simulink library "Snake_Lib"  (R2016a)
settings: Solver=ode45  StartTime=0.0  StopTime=10.0  RelTol=1e-3
libraries: Bit_Demultiplexers_Lib x5, Bit_Multiplexers_Lib x5, simulink_extras x5, commutil2 x2
settings Model: Creator=Jozko Mrkvicka  LastModifiedBy=Jozko Mrkvicka
settings DataIOCC: LimitDataPoints=on
settings DebuggingCC: AllowSymbolicDim=off

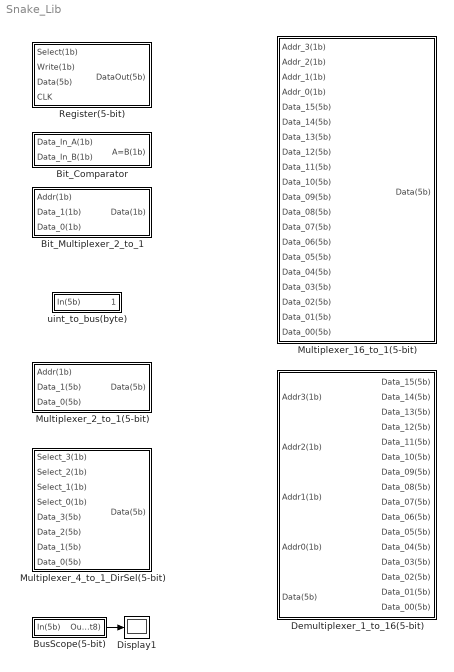
== system Snake_Lib ==
  Bit_Comparator : Subsystem
  Bit_Multiplexer_2_to_1 : Subsystem
  BusScope(5-bit) : Subsystem
  Demultiplexer_1_to_16(5-bit) : Subsystem
  Display1 : Display
  Multiplexer_16_to_1(5-bit) : Subsystem
  Multiplexer_2_to_1(5-bit) : Subsystem
  Multiplexer_4_to_1_DirSel(5-bit) : Subsystem
  Register(5-bit) : Subsystem
  uint_to_bus(byte) : Subsystem
  wires:
  BusScope(5-bit)/1(Out(int8)) -> Display1/1

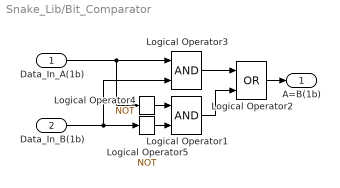
== system Snake_Lib/Bit_Comparator ==
  Data_In_A(1b) : Inport
  Data_In_B(1b) : Inport  Port=2
  Logical Operator1 : Logic  IconShape=distinctive  AllPortsSameDT=off  OutDataTypeStr=boolean
  Logical Operator2 : Logic  Operator=OR  IconShape=distinctive  AllPortsSameDT=off  OutDataTypeStr=boolean
  Logical Operator3 : Logic  IconShape=distinctive  AllPortsSameDT=off  OutDataTypeStr=boolean
  Logical Operator4 : Logic  Operator=NOT  IconShape=distinctive  AllPortsSameDT=off  OutDataTypeStr=boolean
  Logical Operator5 : Logic  Operator=NOT  IconShape=distinctive  AllPortsSameDT=off  OutDataTypeStr=boolean
  A=B(1b) : Outport
  wires:
  Logical Operator4/1 -> Logical Operator1/1
  Logical Operator3/1 -> Logical Operator2/1
  Logical Operator1/1 -> Logical Operator2/2
  Logical Operator2/1 -> A=B(1b)/1
  Data_In_A(1b)/1 -> Logical Operator4/1, Logical Operator3/1
  Logical Operator5/1 -> Logical Operator1/2
  Data_In_B(1b)/1 -> Logical Operator5/1, Logical Operator3/2

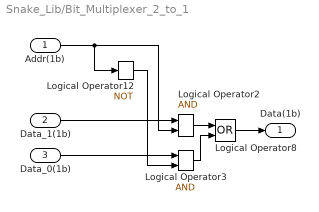
== system Snake_Lib/Bit_Multiplexer_2_to_1 ==
  Addr(1b) : Inport
  Data_1(1b) : Inport  Port=2
  Data_0(1b) : Inport  Port=3
  Logical Operator12 : Logic  Operator=NOT  Inputs=4  IconShape=distinctive  AllPortsSameDT=off  OutDataTypeStr=boolean
  Logical Operator2 : Logic  IconShape=distinctive  AllPortsSameDT=off  OutDataTypeStr=boolean
  Logical Operator3 : Logic  IconShape=distinctive  AllPortsSameDT=off  OutDataTypeStr=boolean
  Logical Operator8 : Logic  Operator=OR  IconShape=distinctive  OutDataTypeStr=boolean
  Data(1b) : Outport
  wires:
  Logical Operator2/1 -> Logical Operator8/1
  Logical Operator3/1 -> Logical Operator8/2
  Data_0(1b)/1 -> Logical Operator3/1
  Data_1(1b)/1 -> Logical Operator2/1
  Logical Operator8/1 -> Data(1b)/1
  Addr(1b)/1 -> Logical Operator12/1, Logical Operator2/2
  Logical Operator12/1 -> Logical Operator3/2

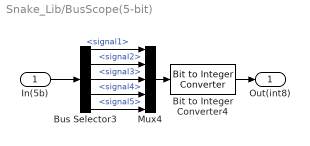
== system Snake_Lib/BusScope(5-bit) ==
  In(5b) : Inport
  Bit to Integer Converter4 : commutil2/Bit to Integer Converter  nbits=5  bitOrder=MSB first  signedOutputValues=Unsigned  outDtype=int8  outDtypeSigned=Inherit via internal rule
  Bus Selector3 : BusSelector  OutputSignals=signal1,signal2,signal3,signal4,signal5
  Mux4 : Mux  Inputs=5
  Out(int8) : Outport
  wires:
  Bus Selector3/2 -> Mux4/2  "<signal2>"
  Bus Selector3/3 -> Mux4/3  "<signal3>"
  Bus Selector3/4 -> Mux4/4  "<signal4>"
  Bus Selector3/5 -> Mux4/5  "<signal5>"
  Bus Selector3/1 -> Mux4/1  "<signal1>"
  Bit to Integer Converter4/1 -> Out(int8)/1
  In(5b)/1 -> Bus Selector3/1
  Mux4/1 -> Bit to Integer Converter4/1

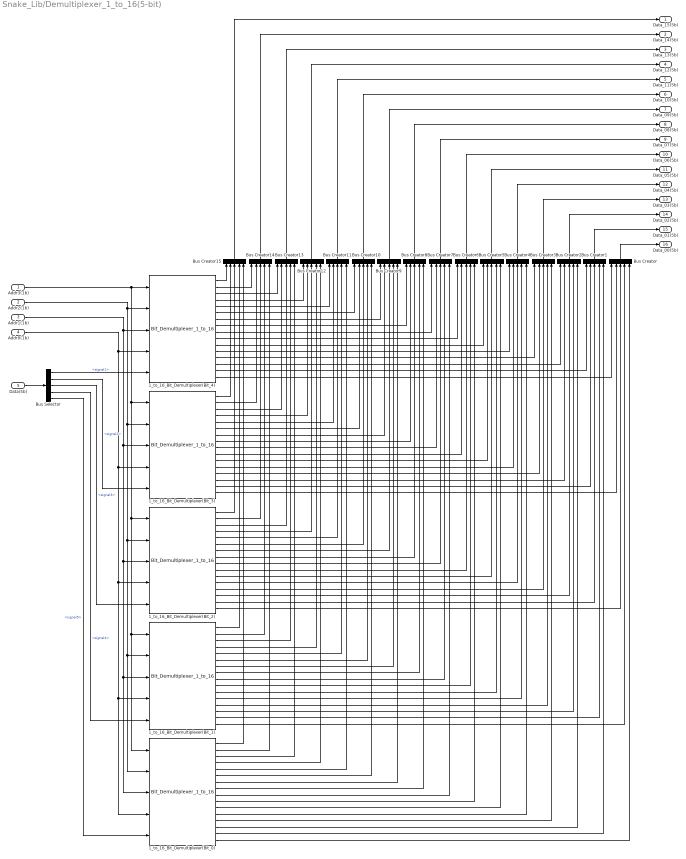
== system Snake_Lib/Demultiplexer_1_to_16(5-bit) ==
  Addr3(1b) : Inport
  Addr2(1b) : Inport  Port=2
  Addr1(1b) : Inport  Port=3
  Addr0(1b) : Inport  Port=4
  Data(5b) : Inport  Port=5
  1_to_16_Bit_Demultiplexer(Bit_0) : Bit_Demultiplexers_Lib/Bit_Demultiplexers_Lib/Bit_Demultiplexer_1_to_16
  1_to_16_Bit_Demultiplexer(Bit_1) : Bit_Demultiplexers_Lib/Bit_Demultiplexers_Lib/Bit_Demultiplexer_1_to_16
  1_to_16_Bit_Demultiplexer(Bit_2) : Bit_Demultiplexers_Lib/Bit_Demultiplexers_Lib/Bit_Demultiplexer_1_to_16
  1_to_16_Bit_Demultiplexer(Bit_3) : Bit_Demultiplexers_Lib/Bit_Demultiplexers_Lib/Bit_Demultiplexer_1_to_16
  1_to_16_Bit_Demultiplexer(Bit_4) : Bit_Demultiplexers_Lib/Bit_Demultiplexers_Lib/Bit_Demultiplexer_1_to_16
  Bus Creator{,1..15} (16 alike) : BusCreator  Inputs=5
  Bus Selector : BusSelector  OutputSignals=signal1,signal2,signal3,signal4,signal5
  Data_15(5b) : Outport
  Data_14(5b) : Outport  Port=2
  Data_13(5b) : Outport  Port=3
  Data_12(5b) : Outport  Port=4
  Data_11(5b) : Outport  Port=5
  Data_10(5b) : Outport  Port=6
  Data_09(5b) : Outport  Port=7
  Data_08(5b) : Outport  Port=8
  Data_07(5b) : Outport  Port=9
  Data_06(5b) : Outport  Port=10
  Data_05(5b) : Outport  Port=11
  Data_04(5b) : Outport  Port=12
  Data_03(5b) : Outport  Port=13
  Data_02(5b) : Outport  Port=14
  Data_01(5b) : Outport  Port=15
  Data_00(5b) : Outport  Port=16
  wires:
  Addr0(1b)/1 -> 1_to_16_Bit_Demultiplexer(Bit_4)/4, 1_to_16_Bit_Demultiplexer(Bit_0)/4, 1_to_16_Bit_Demultiplexer(Bit_1)/4, 1_to_16_Bit_Demultiplexer(Bit_2)/4, 1_to_16_Bit_Demultiplexer(Bit_3)/4
  Addr1(1b)/1 -> 1_to_16_Bit_Demultiplexer(Bit_4)/3, 1_to_16_Bit_Demultiplexer(Bit_0)/3, 1_to_16_Bit_Demultiplexer(Bit_1)/3, 1_to_16_Bit_Demultiplexer(Bit_2)/3, 1_to_16_Bit_Demultiplexer(Bit_3)/3
  Addr2(1b)/1 -> 1_to_16_Bit_Demultiplexer(Bit_4)/2, 1_to_16_Bit_Demultiplexer(Bit_0)/2, 1_to_16_Bit_Demultiplexer(Bit_1)/2, 1_to_16_Bit_Demultiplexer(Bit_2)/2, 1_to_16_Bit_Demultiplexer(Bit_3)/2
  Addr3(1b)/1 -> 1_to_16_Bit_Demultiplexer(Bit_0)/1, 1_to_16_Bit_Demultiplexer(Bit_1)/1, 1_to_16_Bit_Demultiplexer(Bit_2)/1, 1_to_16_Bit_Demultiplexer(Bit_3)/1, 1_to_16_Bit_Demultiplexer(Bit_4)/1
  Data(5b)/1 -> Bus Selector/1
  1_to_16_Bit_Demultiplexer(Bit_4)/1 -> Bus Creator15/1
  1_to_16_Bit_Demultiplexer(Bit_4)/2 -> Bus Creator14/1
  1_to_16_Bit_Demultiplexer(Bit_4)/3 -> Bus Creator13/1
  1_to_16_Bit_Demultiplexer(Bit_4)/4 -> Bus Creator12/1
  1_to_16_Bit_Demultiplexer(Bit_4)/5 -> Bus Creator11/1
  1_to_16_Bit_Demultiplexer(Bit_4)/6 -> Bus Creator10/1
  1_to_16_Bit_Demultiplexer(Bit_4)/7 -> Bus Creator9/1
  1_to_16_Bit_Demultiplexer(Bit_4)/8 -> Bus Creator8/1
  1_to_16_Bit_Demultiplexer(Bit_4)/9 -> Bus Creator7/1
  1_to_16_Bit_Demultiplexer(Bit_4)/10 -> Bus Creator6/1
  1_to_16_Bit_Demultiplexer(Bit_4)/11 -> Bus Creator5/1
  1_to_16_Bit_Demultiplexer(Bit_4)/12 -> Bus Creator4/1
  1_to_16_Bit_Demultiplexer(Bit_4)/13 -> Bus Creator3/1
  1_to_16_Bit_Demultiplexer(Bit_4)/14 -> Bus Creator2/1
  1_to_16_Bit_Demultiplexer(Bit_4)/15 -> Bus Creator1/1
  1_to_16_Bit_Demultiplexer(Bit_4)/16 -> Bus Creator/1
  1_to_16_Bit_Demultiplexer(Bit_3)/1 -> Bus Creator15/2
  1_to_16_Bit_Demultiplexer(Bit_3)/2 -> Bus Creator14/2
  1_to_16_Bit_Demultiplexer(Bit_3)/3 -> Bus Creator13/2
  1_to_16_Bit_Demultiplexer(Bit_3)/4 -> Bus Creator12/2
  1_to_16_Bit_Demultiplexer(Bit_3)/5 -> Bus Creator11/2
  1_to_16_Bit_Demultiplexer(Bit_3)/6 -> Bus Creator10/2
  1_to_16_Bit_Demultiplexer(Bit_3)/7 -> Bus Creator9/2
  1_to_16_Bit_Demultiplexer(Bit_3)/8 -> Bus Creator8/2
  1_to_16_Bit_Demultiplexer(Bit_3)/9 -> Bus Creator7/2
  1_to_16_Bit_Demultiplexer(Bit_3)/10 -> Bus Creator6/2
  1_to_16_Bit_Demultiplexer(Bit_3)/11 -> Bus Creator5/2
  1_to_16_Bit_Demultiplexer(Bit_3)/12 -> Bus Creator4/2
  1_to_16_Bit_Demultiplexer(Bit_3)/13 -> Bus Creator3/2
  1_to_16_Bit_Demultiplexer(Bit_3)/14 -> Bus Creator2/2
  1_to_16_Bit_Demultiplexer(Bit_3)/15 -> Bus Creator1/2
  1_to_16_Bit_Demultiplexer(Bit_3)/16 -> Bus Creator/2
  1_to_16_Bit_Demultiplexer(Bit_2)/1 -> Bus Creator15/3
  1_to_16_Bit_Demultiplexer(Bit_2)/2 -> Bus Creator14/3
  1_to_16_Bit_Demultiplexer(Bit_2)/3 -> Bus Creator13/3
  1_to_16_Bit_Demultiplexer(Bit_2)/4 -> Bus Creator12/3
  1_to_16_Bit_Demultiplexer(Bit_2)/5 -> Bus Creator11/3
  1_to_16_Bit_Demultiplexer(Bit_2)/6 -> Bus Creator10/3
  1_to_16_Bit_Demultiplexer(Bit_2)/7 -> Bus Creator9/3
  1_to_16_Bit_Demultiplexer(Bit_2)/8 -> Bus Creator8/3
  1_to_16_Bit_Demultiplexer(Bit_2)/9 -> Bus Creator7/3
  1_to_16_Bit_Demultiplexer(Bit_2)/10 -> Bus Creator6/3
  1_to_16_Bit_Demultiplexer(Bit_2)/11 -> Bus Creator5/3
  1_to_16_Bit_Demultiplexer(Bit_2)/12 -> Bus Creator4/3
  1_to_16_Bit_Demultiplexer(Bit_2)/13 -> Bus Creator3/3
  1_to_16_Bit_Demultiplexer(Bit_2)/14 -> Bus Creator2/3
  1_to_16_Bit_Demultiplexer(Bit_2)/15 -> Bus Creator1/3
  1_to_16_Bit_Demultiplexer(Bit_2)/16 -> Bus Creator/3
  1_to_16_Bit_Demultiplexer(Bit_1)/1 -> Bus Creator15/4
  1_to_16_Bit_Demultiplexer(Bit_1)/2 -> Bus Creator14/4
  1_to_16_Bit_Demultiplexer(Bit_1)/3 -> Bus Creator13/4
  1_to_16_Bit_Demultiplexer(Bit_1)/4 -> Bus Creator12/4
  1_to_16_Bit_Demultiplexer(Bit_1)/5 -> Bus Creator11/4
  1_to_16_Bit_Demultiplexer(Bit_1)/6 -> Bus Creator10/4
  1_to_16_Bit_Demultiplexer(Bit_1)/7 -> Bus Creator9/4
  1_to_16_Bit_Demultiplexer(Bit_1)/8 -> Bus Creator8/4
  1_to_16_Bit_Demultiplexer(Bit_1)/9 -> Bus Creator7/4
  1_to_16_Bit_Demultiplexer(Bit_1)/10 -> Bus Creator6/4
  1_to_16_Bit_Demultiplexer(Bit_1)/11 -> Bus Creator5/4
  1_to_16_Bit_Demultiplexer(Bit_1)/12 -> Bus Creator4/4
  1_to_16_Bit_Demultiplexer(Bit_1)/13 -> Bus Creator3/4
  1_to_16_Bit_Demultiplexer(Bit_1)/14 -> Bus Creator2/4
  1_to_16_Bit_Demultiplexer(Bit_1)/15 -> Bus Creator1/4
  1_to_16_Bit_Demultiplexer(Bit_1)/16 -> Bus Creator/4
  1_to_16_Bit_Demultiplexer(Bit_0)/1 -> Bus Creator15/5
  1_to_16_Bit_Demultiplexer(Bit_0)/2 -> Bus Creator14/5
  1_to_16_Bit_Demultiplexer(Bit_0)/3 -> Bus Creator13/5
  1_to_16_Bit_Demultiplexer(Bit_0)/4 -> Bus Creator12/5
  1_to_16_Bit_Demultiplexer(Bit_0)/5 -> Bus Creator11/5
  1_to_16_Bit_Demultiplexer(Bit_0)/6 -> Bus Creator10/5
  1_to_16_Bit_Demultiplexer(Bit_0)/7 -> Bus Creator9/5
  1_to_16_Bit_Demultiplexer(Bit_0)/8 -> Bus Creator8/5
  1_to_16_Bit_Demultiplexer(Bit_0)/9 -> Bus Creator7/5
  1_to_16_Bit_Demultiplexer(Bit_0)/10 -> Bus Creator6/5
  1_to_16_Bit_Demultiplexer(Bit_0)/11 -> Bus Creator5/5
  1_to_16_Bit_Demultiplexer(Bit_0)/12 -> Bus Creator4/5
  1_to_16_Bit_Demultiplexer(Bit_0)/13 -> Bus Creator3/5
  1_to_16_Bit_Demultiplexer(Bit_0)/14 -> Bus Creator2/5
  1_to_16_Bit_Demultiplexer(Bit_0)/15 -> Bus Creator1/5
  1_to_16_Bit_Demultiplexer(Bit_0)/16 -> Bus Creator/5
  Bus Creator/1 -> Data_00(5b)/1
  Bus Creator1/1 -> Data_01(5b)/1
  Bus Creator2/1 -> Data_02(5b)/1
  Bus Creator3/1 -> Data_03(5b)/1
  Bus Creator4/1 -> Data_04(5b)/1
  Bus Creator5/1 -> Data_05(5b)/1
  Bus Creator6/1 -> Data_06(5b)/1
  Bus Creator7/1 -> Data_07(5b)/1
  Bus Creator8/1 -> Data_08(5b)/1
  Bus Creator9/1 -> Data_09(5b)/1
  Bus Creator10/1 -> Data_10(5b)/1
  Bus Creator11/1 -> Data_11(5b)/1
  Bus Creator12/1 -> Data_12(5b)/1
  Bus Creator13/1 -> Data_13(5b)/1
  Bus Creator14/1 -> Data_14(5b)/1
  Bus Creator15/1 -> Data_15(5b)/1
  Bus Selector/1 -> 1_to_16_Bit_Demultiplexer(Bit_4)/5  "<signal1>"
  Bus Selector/2 -> 1_to_16_Bit_Demultiplexer(Bit_3)/5  "<signal2>"
  Bus Selector/3 -> 1_to_16_Bit_Demultiplexer(Bit_2)/5  "<signal3>"
  Bus Selector/5 -> 1_to_16_Bit_Demultiplexer(Bit_0)/5  "<signal5>"
  Bus Selector/4 -> 1_to_16_Bit_Demultiplexer(Bit_1)/5  "<signal4>"

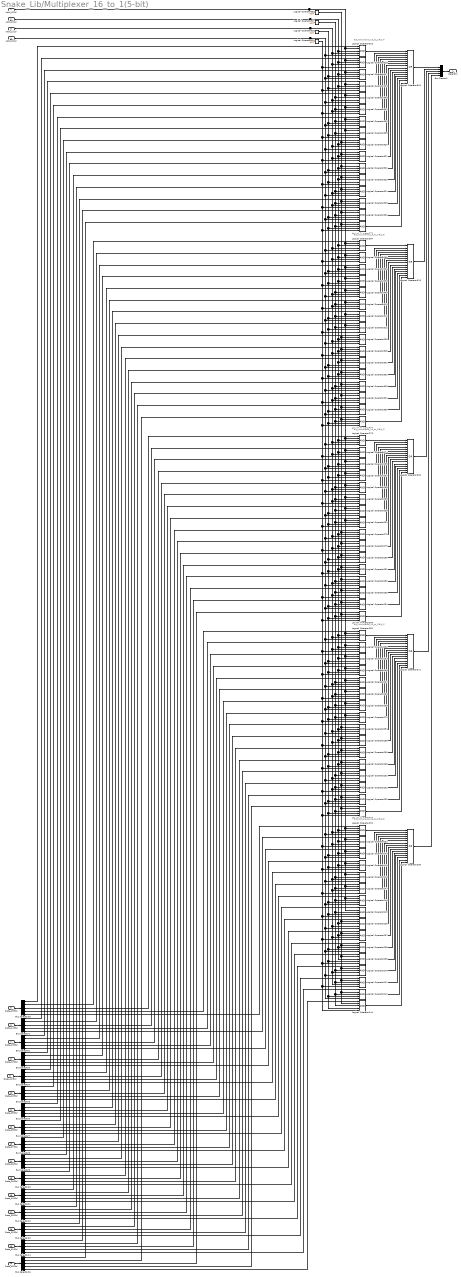
== system Snake_Lib/Multiplexer_16_to_1(5-bit) ==
  note: Bit_Multiplexer_16_to_1(Bit_0)
  note: Bit_Multiplexer_16_to_1(Bit_1)
  note: Bit_Multiplexer_16_to_1(Bit_2)
  note: Bit_Multiplexer_16_to_1(Bit_3)
  note: Bit_Multiplexer_16_to_1(Bit_4)
  Addr_3(1b) : Inport
  Addr_2(1b) : Inport  Port=2
  Addr_1(1b) : Inport  Port=3
  Addr_0(1b) : Inport  Port=4
  Data_15(5b) : Inport  Port=5
  Data_14(5b) : Inport  Port=6
  Data_13(5b) : Inport  Port=7
  Data_12(5b) : Inport  Port=8
  Data_11(5b) : Inport  Port=9
  Data_10(5b) : Inport  Port=10
  Data_09(5b) : Inport  Port=11
  Data_08(5b) : Inport  Port=12
  Data_07(5b) : Inport  Port=13
  Data_06(5b) : Inport  Port=14
  Data_05(5b) : Inport  Port=15
  Data_04(5b) : Inport  Port=16
  Data_03(5b) : Inport  Port=17
  Data_02(5b) : Inport  Port=18
  Data_01(5b) : Inport  Port=19
  Data_00(5b) : Inport  Port=20
  Bus Creator1 : BusCreator  Inputs=5
  Bus Selector{1..16} (16 alike) : BusSelector  OutputSignals=signal1,signal2,signal3,signal4,signal5
  Logical Operator{231..232,236..249,252..253,257..270,273..274,278..291,294..295,299..312,315..316,320..333} (80 alike) : Logic  Inputs=5  IconShape=distinctive  AllPortsSameDT=off  OutDataTypeStr=boolean
  Logical Operator{250,271,292,313,334} (5 alike) : Logic  Operator=OR  Inputs=16  IconShape=distinctive  OutDataTypeStr=boolean
  Logical Operator{317..319,335} (4 alike) : Logic  Operator=NOT  Inputs=4  IconShape=distinctive  AllPortsSameDT=off  OutDataTypeStr=boolean
  Data(5b) : Outport
  wires:
  Logical Operator250/1 -> Bus Creator1/5
  Logical Operator271/1 -> Bus Creator1/4
  Logical Operator292/1 -> Bus Creator1/3
  Logical Operator313/1 -> Bus Creator1/2
  Logical Operator334/1 -> Bus Creator1/1
  Logical Operator315/1 -> Logical Operator334/1
  Logical Operator316/1 -> Logical Operator334/2
  Logical Operator327/1 -> Logical Operator334/3
  Logical Operator329/1 -> Logical Operator334/4
  Logical Operator330/1 -> Logical Operator334/5
  Logical Operator331/1 -> Logical Operator334/6
  Logical Operator332/1 -> Logical Operator334/7
  Logical Operator333/1 -> Logical Operator334/8
  Bus Selector7/1 -> Logical Operator333/1  "<signal1>"
  Bus Selector6/1 -> Logical Operator332/1  "<signal1>"
  Bus Selector5/1 -> Logical Operator331/1  "<signal1>"
  Bus Selector4/1 -> Logical Operator330/1  "<signal1>"
  Bus Selector3/1 -> Logical Operator329/1  "<signal1>"
  Bus Selector2/1 -> Logical Operator327/1  "<signal1>"
  Bus Selector1/1 -> Logical Operator316/1  "<signal1>"
  Bus Selector15/1 -> Logical Operator315/1  "<signal1>"
  Logical Operator320/1 -> Logical Operator334/9
  Logical Operator321/1 -> Logical Operator334/10
  Logical Operator322/1 -> Logical Operator334/11
  Logical Operator323/1 -> Logical Operator334/12
  Logical Operator324/1 -> Logical Operator334/13
  Logical Operator325/1 -> Logical Operator334/14
  Logical Operator326/1 -> Logical Operator334/15
  Logical Operator328/1 -> Logical Operator334/16
  Bus Selector8/1 -> Logical Operator320/1  "<signal1>"
  Bus Selector9/1 -> Logical Operator321/1  "<signal1>"
  Bus Selector10/1 -> Logical Operator322/1  "<signal1>"
  Bus Selector11/1 -> Logical Operator323/1  "<signal1>"
  Bus Selector12/1 -> Logical Operator324/1  "<signal1>"
  Bus Selector13/1 -> Logical Operator325/1  "<signal1>"
  Bus Selector14/1 -> Logical Operator326/1  "<signal1>"
  Bus Selector16/1 -> Logical Operator328/1  "<signal1>"
  Addr_3(1b)/1 -> Logical Operator315/2, Logical Operator316/2, Logical Operator327/2, Logical Operator329/2, Logical Operator330/2, Logical Operator331/2, Logical Operator332/2, Logical Operator333/2, Logical Operator294/2, Logical Operator295/2, Logical Operator306/2, Logical Operator308/2, Logical Operator309/2, Logical Operator310/2, Logical Operator311/2, Logical Operator312/2, Logical Operator273/2, Logical Operator274/2, Logical Operator285/2, Logical Operator287/2, Logical Operator288/2, Logical Operator289/2, Logical Operator290/2, Logical Operator291/2, Logical Operator252/2, Logical Operator253/2, Logical Operator264/2, Logical Operator266/2, Logical Operator267/2, Logical Operator268/2, Logical Operator269/2, Logical Operator270/2, Logical Operator231/2, Logical Operator232/2, Logical Operator243/2, Logical Operator245/2, Logical Operator246/2, Logical Operator247/2, Logical Operator248/2, Logical Operator249/2, Logical Operator335/1
  Addr_2(1b)/1 -> Logical Operator315/3, Logical Operator316/3, Logical Operator327/3, Logical Operator329/3, Logical Operator320/3, Logical Operator321/3, Logical Operator322/3, Logical Operator323/3, Logical Operator294/3, Logical Operator295/3, Logical Operator306/3, Logical Operator308/3, Logical Operator299/3, Logical Operator300/3, Logical Operator301/3, Logical Operator302/3, Logical Operator273/3, Logical Operator274/3, Logical Operator285/3, Logical Operator287/3, Logical Operator278/3, Logical Operator279/3, Logical Operator280/3, Logical Operator281/3, Logical Operator252/3, Logical Operator253/3, Logical Operator264/3, Logical Operator266/3, Logical Operator257/3, Logical Operator258/3, Logical Operator259/3, Logical Operator260/3, Logical Operator231/3, Logical Operator232/3, Logical Operator243/3, Logical Operator245/3, Logical Operator236/3, Logical Operator237/3, Logical Operator238/3, Logical Operator239/3, Logical Operator317/1
  Addr_1(1b)/1 -> Logical Operator315/4, Logical Operator316/4, Logical Operator330/4, Logical Operator331/4, Logical Operator320/4, Logical Operator321/4, Logical Operator324/4, Logical Operator325/4, Logical Operator294/4, Logical Operator295/4, Logical Operator309/4, Logical Operator310/4, Logical Operator299/4, Logical Operator300/4, Logical Operator303/4, Logical Operator304/4, Logical Operator273/4, Logical Operator274/4, Logical Operator288/4, Logical Operator289/4, Logical Operator278/4, Logical Operator279/4, Logical Operator282/4, Logical Operator283/4, Logical Operator252/4, Logical Operator253/4, Logical Operator267/4, Logical Operator268/4, Logical Operator257/4, Logical Operator258/4, Logical Operator261/4, Logical Operator262/4, Logical Operator231/4, Logical Operator232/4, Logical Operator246/4, Logical Operator247/4, Logical Operator236/4, Logical Operator237/4, Logical Operator240/4, Logical Operator241/4, Logical Operator318/1
  Addr_0(1b)/1 -> Logical Operator315/5, Logical Operator327/5, Logical Operator330/5, Logical Operator332/5, Logical Operator320/5, Logical Operator322/5, Logical Operator324/5, Logical Operator326/5, Logical Operator294/5, Logical Operator306/5, Logical Operator309/5, Logical Operator311/5, Logical Operator299/5, Logical Operator301/5, Logical Operator303/5, Logical Operator305/5, Logical Operator273/5, Logical Operator285/5, Logical Operator288/5, Logical Operator290/5, Logical Operator278/5, Logical Operator280/5, Logical Operator282/5, Logical Operator284/5, Logical Operator252/5, Logical Operator264/5, Logical Operator267/5, Logical Operator269/5, Logical Operator257/5, Logical Operator259/5, Logical Operator261/5, Logical Operator263/5, Logical Operator231/5, Logical Operator243/5, Logical Operator246/5, Logical Operator248/5, Logical Operator236/5, Logical Operator238/5, Logical Operator240/5, Logical Operator242/5, Logical Operator319/1
  Logical Operator294/1 -> Logical Operator313/1
  Logical Operator295/1 -> Logical Operator313/2
  Logical Operator306/1 -> Logical Operator313/3
  Logical Operator308/1 -> Logical Operator313/4
  Logical Operator309/1 -> Logical Operator313/5
  Logical Operator310/1 -> Logical Operator313/6
  Logical Operator311/1 -> Logical Operator313/7
  Logical Operator312/1 -> Logical Operator313/8
  Bus Selector7/2 -> Logical Operator312/1  "<signal2>"
  Bus Selector6/2 -> Logical Operator311/1  "<signal2>"
  Bus Selector5/2 -> Logical Operator310/1  "<signal2>"
  Bus Selector4/2 -> Logical Operator309/1  "<signal2>"
  Bus Selector3/2 -> Logical Operator308/1  "<signal2>"
  Bus Selector2/2 -> Logical Operator306/1  "<signal2>"
  Bus Selector1/2 -> Logical Operator295/1  "<signal2>"
  Bus Selector15/2 -> Logical Operator294/1  "<signal2>"
  Logical Operator299/1 -> Logical Operator313/9
  Logical Operator300/1 -> Logical Operator313/10
  Logical Operator301/1 -> Logical Operator313/11
  Logical Operator302/1 -> Logical Operator313/12
  Logical Operator303/1 -> Logical Operator313/13
  Logical Operator304/1 -> Logical Operator313/14
  Logical Operator305/1 -> Logical Operator313/15
  Logical Operator307/1 -> Logical Operator313/16
  Bus Selector8/2 -> Logical Operator299/1  "<signal2>"
  Bus Selector9/2 -> Logical Operator300/1  "<signal2>"
  Bus Selector10/2 -> Logical Operator301/1  "<signal2>"
  Bus Selector11/2 -> Logical Operator302/1  "<signal2>"
  Bus Selector12/2 -> Logical Operator303/1  "<signal2>"
  Bus Selector13/2 -> Logical Operator304/1  "<signal2>"
  Bus Selector14/2 -> Logical Operator305/1  "<signal2>"
  Bus Selector16/2 -> Logical Operator307/1  "<signal2>"
  Logical Operator273/1 -> Logical Operator292/1
  Logical Operator274/1 -> Logical Operator292/2
  Logical Operator285/1 -> Logical Operator292/3
  Logical Operator287/1 -> Logical Operator292/4
  Logical Operator288/1 -> Logical Operator292/5
  Logical Operator289/1 -> Logical Operator292/6
  Logical Operator290/1 -> Logical Operator292/7
  Logical Operator291/1 -> Logical Operator292/8
  Bus Selector7/3 -> Logical Operator291/1  "<signal3>"
  Bus Selector6/3 -> Logical Operator290/1  "<signal3>"
  Bus Selector5/3 -> Logical Operator289/1  "<signal3>"
  Bus Selector4/3 -> Logical Operator288/1  "<signal3>"
  Bus Selector3/3 -> Logical Operator287/1  "<signal3>"
  Bus Selector2/3 -> Logical Operator285/1  "<signal3>"
  Bus Selector1/3 -> Logical Operator274/1  "<signal3>"
  Bus Selector15/3 -> Logical Operator273/1  "<signal3>"
  Logical Operator278/1 -> Logical Operator292/9
  Logical Operator279/1 -> Logical Operator292/10
  Logical Operator280/1 -> Logical Operator292/11
  Logical Operator281/1 -> Logical Operator292/12
  Logical Operator282/1 -> Logical Operator292/13
  Logical Operator283/1 -> Logical Operator292/14
  Logical Operator284/1 -> Logical Operator292/15
  Logical Operator286/1 -> Logical Operator292/16
  Bus Selector8/3 -> Logical Operator278/1  "<signal3>"
  Bus Selector9/3 -> Logical Operator279/1  "<signal3>"
  Bus Selector10/3 -> Logical Operator280/1  "<signal3>"
  Bus Selector11/3 -> Logical Operator281/1  "<signal3>"
  Bus Selector12/3 -> Logical Operator282/1  "<signal3>"
  Bus Selector13/3 -> Logical Operator283/1  "<signal3>"
  Bus Selector14/3 -> Logical Operator284/1  "<signal3>"
  Bus Selector16/3 -> Logical Operator286/1  "<signal3>"
  Logical Operator252/1 -> Logical Operator271/1
  Logical Operator253/1 -> Logical Operator271/2
  Logical Operator264/1 -> Logical Operator271/3
  Logical Operator266/1 -> Logical Operator271/4
  Logical Operator267/1 -> Logical Operator271/5
  Logical Operator268/1 -> Logical Operator271/6
  Logical Operator269/1 -> Logical Operator271/7
  Logical Operator270/1 -> Logical Operator271/8
  Bus Selector7/4 -> Logical Operator270/1  "<signal4>"
  Bus Selector6/4 -> Logical Operator269/1  "<signal4>"
  Bus Selector5/4 -> Logical Operator268/1  "<signal4>"
  Bus Selector4/4 -> Logical Operator267/1  "<signal4>"
  Bus Selector3/4 -> Logical Operator266/1  "<signal4>"
  Bus Selector2/4 -> Logical Operator264/1  "<signal4>"
  Bus Selector1/4 -> Logical Operator253/1  "<signal4>"
  Bus Selector15/4 -> Logical Operator252/1  "<signal4>"
  Logical Operator257/1 -> Logical Operator271/9
  Logical Operator258/1 -> Logical Operator271/10
  Logical Operator259/1 -> Logical Operator271/11
  Logical Operator260/1 -> Logical Operator271/12
  Logical Operator261/1 -> Logical Operator271/13
  Logical Operator262/1 -> Logical Operator271/14
  Logical Operator263/1 -> Logical Operator271/15
  Logical Operator265/1 -> Logical Operator271/16
  Bus Selector8/4 -> Logical Operator257/1  "<signal4>"
  Bus Selector9/4 -> Logical Operator258/1  "<signal4>"
  Bus Selector10/4 -> Logical Operator259/1  "<signal4>"
  Bus Selector11/4 -> Logical Operator260/1  "<signal4>"
  Bus Selector12/4 -> Logical Operator261/1  "<signal4>"
  Bus Selector13/4 -> Logical Operator262/1  "<signal4>"
  Bus Selector14/4 -> Logical Operator263/1  "<signal4>"
  Bus Selector16/4 -> Logical Operator265/1  "<signal4>"
  Logical Operator231/1 -> Logical Operator250/1
  Logical Operator232/1 -> Logical Operator250/2
  Logical Operator243/1 -> Logical Operator250/3
  Logical Operator245/1 -> Logical Operator250/4
  Logical Operator246/1 -> Logical Operator250/5
  Logical Operator247/1 -> Logical Operator250/6
  Logical Operator248/1 -> Logical Operator250/7
  Logical Operator249/1 -> Logical Operator250/8
  Bus Selector7/5 -> Logical Operator249/1  "<signal5>"
  Bus Selector6/5 -> Logical Operator248/1  "<signal5>"
  Bus Selector5/5 -> Logical Operator247/1  "<signal5>"
  Bus Selector4/5 -> Logical Operator246/1  "<signal5>"
  Bus Selector3/5 -> Logical Operator245/1  "<signal5>"
  Bus Selector2/5 -> Logical Operator243/1  "<signal5>"
  Bus Selector1/5 -> Logical Operator232/1  "<signal5>"
  Bus Selector15/5 -> Logical Operator231/1  "<signal5>"
  Logical Operator236/1 -> Logical Operator250/9
  Logical Operator237/1 -> Logical Operator250/10
  Logical Operator238/1 -> Logical Operator250/11
  Logical Operator239/1 -> Logical Operator250/12
  Logical Operator240/1 -> Logical Operator250/13
  Logical Operator241/1 -> Logical Operator250/14
  Logical Operator242/1 -> Logical Operator250/15
  Logical Operator244/1 -> Logical Operator250/16
  Bus Selector8/5 -> Logical Operator236/1  "<signal5>"
  Bus Selector9/5 -> Logical Operator237/1  "<signal5>"
  Bus Selector10/5 -> Logical Operator238/1  "<signal5>"
  Bus Selector11/5 -> Logical Operator239/1  "<signal5>"
  Bus Selector12/5 -> Logical Operator240/1  "<signal5>"
  Bus Selector13/5 -> Logical Operator241/1  "<signal5>"
  Bus Selector14/5 -> Logical Operator242/1  "<signal5>"
  Bus Selector16/5 -> Logical Operator244/1  "<signal5>"
  Logical Operator335/1 -> Logical Operator328/2, Logical Operator299/2, Logical Operator300/2, Logical Operator301/2, Logical Operator302/2, Logical Operator303/2, Logical Operator304/2, Logical Operator305/2, Logical Operator307/2, Logical Operator278/2, Logical Operator279/2, Logical Operator280/2, Logical Operator281/2, Logical Operator282/2, Logical Operator283/2, Logical Operator284/2, Logical Operator286/2, Logical Operator257/2, Logical Operator258/2, Logical Operator259/2, Logical Operator260/2, Logical Operator261/2, Logical Operator262/2, Logical Operator263/2, Logical Operator265/2, Logical Operator236/2, Logical Operator237/2, Logical Operator238/2, Logical Operator239/2, Logical Operator240/2, Logical Operator241/2, Logical Operator242/2, Logical Operator244/2, Logical Operator326/2, Logical Operator325/2, Logical Operator324/2, Logical Operator323/2, Logical Operator322/2, Logical Operator321/2, Logical Operator320/2
  Logical Operator317/1 -> Logical Operator328/3, Logical Operator309/3, Logical Operator310/3, Logical Operator311/3, Logical Operator312/3, Logical Operator303/3, Logical Operator304/3, Logical Operator305/3, Logical Operator307/3, Logical Operator288/3, Logical Operator289/3, Logical Operator290/3, Logical Operator291/3, Logical Operator282/3, Logical Operator283/3, Logical Operator284/3, Logical Operator286/3, Logical Operator267/3, Logical Operator268/3, Logical Operator269/3, Logical Operator270/3, Logical Operator261/3, Logical Operator262/3, Logical Operator263/3, Logical Operator265/3, Logical Operator246/3, Logical Operator247/3, Logical Operator248/3, Logical Operator249/3, Logical Operator240/3, Logical Operator241/3, Logical Operator242/3, Logical Operator244/3, Logical Operator326/3, Logical Operator325/3, Logical Operator324/3, Logical Operator333/3, Logical Operator332/3, Logical Operator331/3, Logical Operator330/3
  Logical Operator318/1 -> Logical Operator328/4, Logical Operator306/4, Logical Operator308/4, Logical Operator311/4, Logical Operator312/4, Logical Operator301/4, Logical Operator302/4, Logical Operator305/4, Logical Operator307/4, Logical Operator285/4, Logical Operator287/4, Logical Operator290/4, Logical Operator291/4, Logical Operator280/4, Logical Operator281/4, Logical Operator284/4, Logical Operator286/4, Logical Operator264/4, Logical Operator266/4, Logical Operator269/4, Logical Operator270/4, Logical Operator259/4, Logical Operator260/4, Logical Operator263/4, Logical Operator265/4, Logical Operator243/4, Logical Operator245/4, Logical Operator248/4, Logical Operator249/4, Logical Operator238/4, Logical Operator239/4, Logical Operator242/4, Logical Operator244/4, Logical Operator326/4, Logical Operator323/4, Logical Operator322/4, Logical Operator333/4, Logical Operator332/4, Logical Operator329/4, Logical Operator327/4
  Logical Operator319/1 -> Logical Operator316/5, Logical Operator328/5, Logical Operator295/5, Logical Operator308/5, Logical Operator310/5, Logical Operator312/5, Logical Operator300/5, Logical Operator302/5, Logical Operator304/5, Logical Operator307/5, Logical Operator274/5, Logical Operator287/5, Logical Operator289/5, Logical Operator291/5, Logical Operator279/5, Logical Operator281/5, Logical Operator283/5, Logical Operator286/5, Logical Operator253/5, Logical Operator266/5, Logical Operator268/5, Logical Operator270/5, Logical Operator258/5, Logical Operator260/5, Logical Operator262/5, Logical Operator265/5, Logical Operator232/5, Logical Operator245/5, Logical Operator247/5, Logical Operator249/5, Logical Operator237/5, Logical Operator239/5, Logical Operator241/5, Logical Operator244/5, Logical Operator325/5, Logical Operator323/5, Logical Operator321/5, Logical Operator333/5, Logical Operator331/5, Logical Operator329/5
  Bus Creator1/1 -> Data(5b)/1
  Data_00(5b)/1 -> Bus Selector16/1
  Data_01(5b)/1 -> Bus Selector14/1
  Data_02(5b)/1 -> Bus Selector13/1
  Data_03(5b)/1 -> Bus Selector12/1
  Data_04(5b)/1 -> Bus Selector11/1
  Data_05(5b)/1 -> Bus Selector10/1
  Data_06(5b)/1 -> Bus Selector9/1
  Data_07(5b)/1 -> Bus Selector8/1
  Data_08(5b)/1 -> Bus Selector7/1
  Data_09(5b)/1 -> Bus Selector6/1
  Data_10(5b)/1 -> Bus Selector5/1
  Data_11(5b)/1 -> Bus Selector4/1
  Data_12(5b)/1 -> Bus Selector3/1
  Data_13(5b)/1 -> Bus Selector2/1
  Data_14(5b)/1 -> Bus Selector1/1
  Data_15(5b)/1 -> Bus Selector15/1

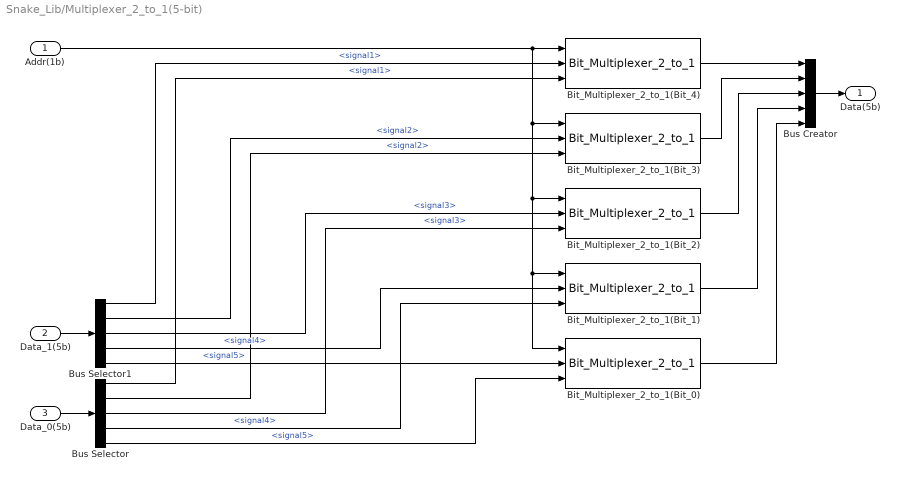
== system Snake_Lib/Multiplexer_2_to_1(5-bit) ==
  Addr(1b) : Inport
  Data_1(5b) : Inport  Port=2
  Data_0(5b) : Inport  Port=3
  Bit_Multiplexer_2_to_1(Bit_0) : Bit_Multiplexers_Lib/Bit_Multiplexers_Lib/Bit_Multiplexer_2_to_1
  Bit_Multiplexer_2_to_1(Bit_1) : Bit_Multiplexers_Lib/Bit_Multiplexers_Lib/Bit_Multiplexer_2_to_1
  Bit_Multiplexer_2_to_1(Bit_2) : Bit_Multiplexers_Lib/Bit_Multiplexers_Lib/Bit_Multiplexer_2_to_1
  Bit_Multiplexer_2_to_1(Bit_3) : Bit_Multiplexers_Lib/Bit_Multiplexers_Lib/Bit_Multiplexer_2_to_1
  Bit_Multiplexer_2_to_1(Bit_4) : Bit_Multiplexers_Lib/Bit_Multiplexers_Lib/Bit_Multiplexer_2_to_1
  Bus Creator : BusCreator  Inputs=5
  Bus Selector : BusSelector  OutputSignals=signal1,signal2,signal3,signal4,signal5
  Bus Selector1 : BusSelector  OutputSignals=signal1,signal2,signal3,signal4,signal5
  Data(5b) : Outport
  wires:
  Bus Selector1/1 -> Bit_Multiplexer_2_to_1(Bit_4)/2  "<signal1>"
  Bus Selector/1 -> Bit_Multiplexer_2_to_1(Bit_4)/3  "<signal1>"
  Bus Selector/2 -> Bit_Multiplexer_2_to_1(Bit_3)/3  "<signal2>"
  Bus Selector1/2 -> Bit_Multiplexer_2_to_1(Bit_3)/2  "<signal2>"
  Bus Selector/3 -> Bit_Multiplexer_2_to_1(Bit_2)/3  "<signal3>"
  Bus Selector1/3 -> Bit_Multiplexer_2_to_1(Bit_2)/2  "<signal3>"
  Bus Selector1/4 -> Bit_Multiplexer_2_to_1(Bit_1)/2  "<signal4>"
  Bus Selector/4 -> Bit_Multiplexer_2_to_1(Bit_1)/3  "<signal4>"
  Bus Selector1/5 -> Bit_Multiplexer_2_to_1(Bit_0)/2  "<signal5>"
  Bus Selector/5 -> Bit_Multiplexer_2_to_1(Bit_0)/3  "<signal5>"
  Data_0(5b)/1 -> Bus Selector/1
  Data_1(5b)/1 -> Bus Selector1/1
  Bit_Multiplexer_2_to_1(Bit_0)/1 -> Bus Creator/5
  Bit_Multiplexer_2_to_1(Bit_4)/1 -> Bus Creator/1
  Bit_Multiplexer_2_to_1(Bit_3)/1 -> Bus Creator/2
  Bit_Multiplexer_2_to_1(Bit_2)/1 -> Bus Creator/3
  Bit_Multiplexer_2_to_1(Bit_1)/1 -> Bus Creator/4
  Addr(1b)/1 -> Bit_Multiplexer_2_to_1(Bit_3)/1, Bit_Multiplexer_2_to_1(Bit_2)/1, Bit_Multiplexer_2_to_1(Bit_1)/1, Bit_Multiplexer_2_to_1(Bit_0)/1, Bit_Multiplexer_2_to_1(Bit_4)/1
  Bus Creator/1 -> Data(5b)/1

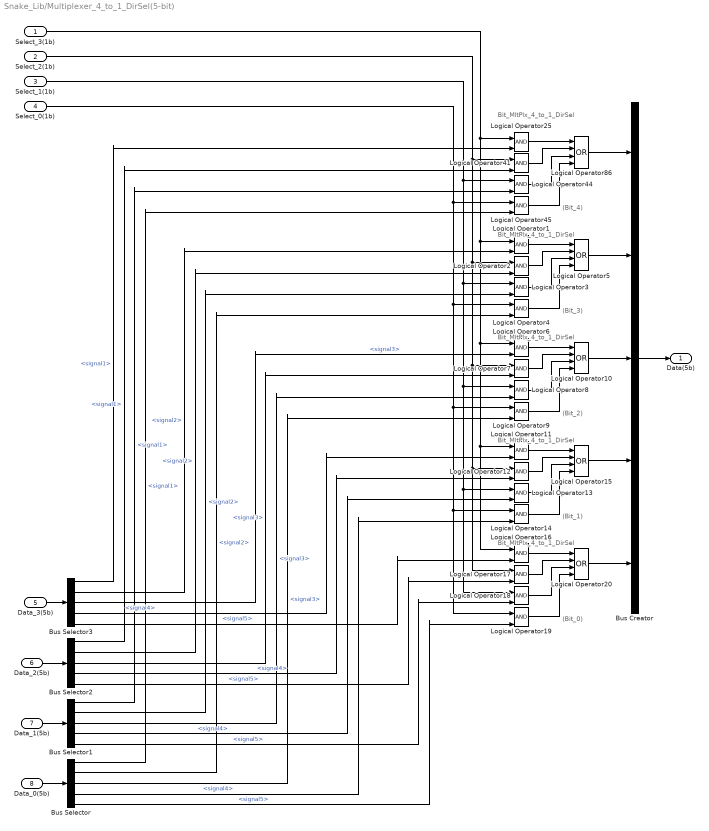
== system Snake_Lib/Multiplexer_4_to_1_DirSel(5-bit) ==
  note: Bit_MltPlx_4_to_1_DirSel
  note: (Bit_0)
  note: Bit_MltPlx_4_to_1_DirSel
  note: (Bit_1)
  note: Bit_MltPlx_4_to_1_DirSel
  note: (Bit_2)
  note: Bit_MltPlx_4_to_1_DirSel
  note: (Bit_3)
  note: Bit_MltPlx_4_to_1_DirSel
  note: (Bit_4)
  Select_3(1b) : Inport
  Select_2(1b) : Inport  Port=2
  Select_1(1b) : Inport  Port=3
  Select_0(1b) : Inport  Port=4
  Data_3(5b) : Inport  Port=5
  Data_2(5b) : Inport  Port=6
  Data_1(5b) : Inport  Port=7
  Data_0(5b) : Inport  Port=8
  Bus Creator : BusCreator  Inputs=5
  Bus Selector{,1..3} (4 alike) : BusSelector  OutputSignals=signal1,signal2,signal3,signal4,signal5
  Logical Operator{1..4,6..9,11..14,16..19,25,41,44..45} (20 alike) : Logic  IconShape=distinctive  AllPortsSameDT=off  OutDataTypeStr=boolean
  Logical Operator{5,10,15,20,86} (5 alike) : Logic  Operator=OR  Inputs=4  IconShape=distinctive  OutDataTypeStr=boolean
  Data(5b) : Outport
  wires:
  Logical Operator16/1 -> Logical Operator20/1
  Logical Operator17/1 -> Logical Operator20/2
  Logical Operator18/1 -> Logical Operator20/3
  Logical Operator19/1 -> Logical Operator20/4
  Logical Operator11/1 -> Logical Operator15/1
  Logical Operator12/1 -> Logical Operator15/2
  Logical Operator13/1 -> Logical Operator15/3
  Logical Operator14/1 -> Logical Operator15/4
  Logical Operator6/1 -> Logical Operator10/1
  Logical Operator7/1 -> Logical Operator10/2
  Logical Operator8/1 -> Logical Operator10/3
  Logical Operator9/1 -> Logical Operator10/4
  Logical Operator1/1 -> Logical Operator5/1
  Logical Operator2/1 -> Logical Operator5/2
  Logical Operator3/1 -> Logical Operator5/3
  Logical Operator4/1 -> Logical Operator5/4
  Logical Operator20/1 -> Bus Creator/5
  Logical Operator15/1 -> Bus Creator/4
  Logical Operator10/1 -> Bus Creator/3
  Logical Operator5/1 -> Bus Creator/2
  Select_1(1b)/1 -> Logical Operator44/1, Logical Operator3/1, Logical Operator8/1, Logical Operator13/1, Logical Operator18/1
  Select_0(1b)/1 -> Logical Operator45/1, Logical Operator4/1, Logical Operator9/1, Logical Operator14/1, Logical Operator19/1
  Select_2(1b)/1 -> Logical Operator41/1, Logical Operator2/1, Logical Operator7/1, Logical Operator12/1, Logical Operator17/1
  Select_3(1b)/1 -> Logical Operator25/1, Logical Operator1/1, Logical Operator16/1, Logical Operator11/1, Logical Operator6/1
  Logical Operator25/1 -> Logical Operator86/1
  Logical Operator41/1 -> Logical Operator86/2
  Logical Operator44/1 -> Logical Operator86/3
  Logical Operator45/1 -> Logical Operator86/4
  Logical Operator86/1 -> Bus Creator/1
  Bus Selector3/1 -> Logical Operator25/2  "<signal1>"
  Bus Selector2/1 -> Logical Operator41/2  "<signal1>"
  Bus Selector1/1 -> Logical Operator44/2  "<signal1>"
  Bus Selector/1 -> Logical Operator45/2  "<signal1>"
  Bus Selector3/2 -> Logical Operator1/2  "<signal2>"
  Bus Selector2/2 -> Logical Operator2/2  "<signal2>"
  Bus Selector1/2 -> Logical Operator3/2  "<signal2>"
  Bus Selector/2 -> Logical Operator4/2  "<signal2>"
  Bus Selector3/3 -> Logical Operator6/2  "<signal3>"
  Bus Selector2/3 -> Logical Operator7/2  "<signal3>"
  Bus Selector1/3 -> Logical Operator8/2  "<signal3>"
  Bus Selector/3 -> Logical Operator9/2  "<signal3>"
  Bus Selector3/4 -> Logical Operator11/2  "<signal4>"
  Bus Selector2/4 -> Logical Operator12/2  "<signal4>"
  Bus Selector1/4 -> Logical Operator13/2  "<signal4>"
  Bus Selector/4 -> Logical Operator14/2  "<signal4>"
  Bus Selector3/5 -> Logical Operator16/2  "<signal5>"
  Bus Selector2/5 -> Logical Operator17/2  "<signal5>"
  Bus Selector1/5 -> Logical Operator18/2  "<signal5>"
  Bus Selector/5 -> Logical Operator19/2  "<signal5>"
  Bus Creator/1 -> Data(5b)/1
  Data_0(5b)/1 -> Bus Selector/1
  Data_1(5b)/1 -> Bus Selector1/1
  Data_2(5b)/1 -> Bus Selector2/1
  Data_3(5b)/1 -> Bus Selector3/1

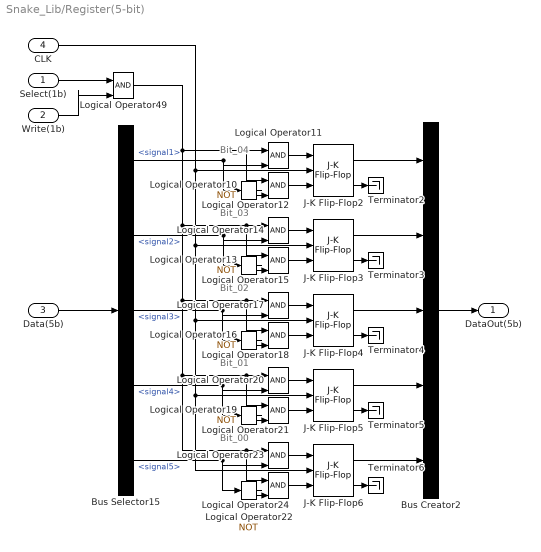
== system Snake_Lib/Register(5-bit) ==
  note: Bit_00
  note: Bit_01
  note: Bit_02
  note: Bit_03
  note: Bit_04
  Select(1b) : Inport
  Write(1b) : Inport  Port=2
  Data(5b) : Inport  Port=3
  CLK : Inport  Port=4  OutDataTypeStr=double
  Bus Creator2 : BusCreator  Inputs=5
  Bus Selector15 : BusSelector  OutputSignals=signal1,signal2,signal3,signal4,signal5
  J-K Flip-Flop{2..6} (5 alike) : simulink_extras/Flip Flops/J-K Flip-Flop  initial_condition=0
  Logical Operator{10,13,16,19,22} (5 alike) : Logic  Operator=NOT  IconShape=distinctive  AllPortsSameDT=off  OutDataTypeStr=boolean
  Logical Operator{11..12,14..15,17..18,20..21,23..24,49} (11 alike) : Logic  IconShape=distinctive  AllPortsSameDT=off  OutDataTypeStr=boolean
  Terminator{2..6} (5 alike) : Terminator
  DataOut(5b) : Outport
  wires:
  Bus Creator2/1 -> DataOut(5b)/1
  Bus Selector15/5 -> Logical Operator22/1, Logical Operator23/2  "<signal5>"
  J-K Flip-Flop6/2 -> Terminator6/1
  J-K Flip-Flop6/1 -> Bus Creator2/5
  Logical Operator22/1 -> Logical Operator24/2
  Logical Operator23/1 -> J-K Flip-Flop6/1
  Logical Operator24/1 -> J-K Flip-Flop6/3
  Bus Selector15/4 -> Logical Operator19/1, Logical Operator20/2  "<signal4>"
  J-K Flip-Flop5/2 -> Terminator5/1
  J-K Flip-Flop5/1 -> Bus Creator2/4
  Logical Operator49/1 -> Logical Operator20/1, Logical Operator21/1, Logical Operator23/1, Logical Operator24/1, Logical Operator17/1, Logical Operator18/1, Logical Operator14/1, Logical Operator15/1, Logical Operator11/1, Logical Operator12/1
  Logical Operator19/1 -> Logical Operator21/2
  Logical Operator20/1 -> J-K Flip-Flop5/1
  Logical Operator21/1 -> J-K Flip-Flop5/3
  Bus Selector15/3 -> Logical Operator17/2, Logical Operator16/1  "<signal3>"
  J-K Flip-Flop4/2 -> Terminator4/1
  J-K Flip-Flop4/1 -> Bus Creator2/3
  Logical Operator16/1 -> Logical Operator18/2
  Logical Operator17/1 -> J-K Flip-Flop4/1
  Logical Operator18/1 -> J-K Flip-Flop4/3
  Bus Selector15/2 -> Logical Operator14/2, Logical Operator13/1  "<signal2>"
  J-K Flip-Flop3/2 -> Terminator3/1
  J-K Flip-Flop3/1 -> Bus Creator2/2
  Logical Operator13/1 -> Logical Operator15/2
  Logical Operator14/1 -> J-K Flip-Flop3/1
  Logical Operator15/1 -> J-K Flip-Flop3/3
  Bus Selector15/1 -> Logical Operator10/1, Logical Operator11/2  "<signal1>"
  J-K Flip-Flop2/2 -> Terminator2/1
  J-K Flip-Flop2/1 -> Bus Creator2/1
  Logical Operator10/1 -> Logical Operator12/2
  Logical Operator11/1 -> J-K Flip-Flop2/1
  Logical Operator12/1 -> J-K Flip-Flop2/3
  CLK/1 -> J-K Flip-Flop2/2, J-K Flip-Flop3/2, J-K Flip-Flop4/2, J-K Flip-Flop5/2, J-K Flip-Flop6/2
  Data(5b)/1 -> Bus Selector15/1
  Select(1b)/1 -> Logical Operator49/1
  Write(1b)/1 -> Logical Operator49/2

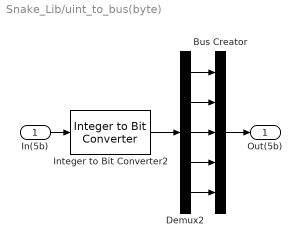
== system Snake_Lib/uint_to_bus(byte) ==
  In(5b) : Inport
  Bus Creator : BusCreator  Inputs=5
  Demux2 : Demux  Outputs=5
  Integer to Bit Converter2 : commutil2/Integer to Bit Converter  nbits=5  signedInputValues=Unsigned  bitOrder=MSB first  outDtype=boolean
  Out(5b) : Outport
  wires:
  Demux2/5 -> Bus Creator/5
  Demux2/4 -> Bus Creator/4
  Demux2/3 -> Bus Creator/3
  Demux2/2 -> Bus Creator/2
  Demux2/1 -> Bus Creator/1
  Integer to Bit Converter2/1 -> Demux2/1
  Bus Creator/1 -> Out(5b)/1
  In(5b)/1 -> Integer to Bit Converter2/1
